simulink model "TPEtape3simulink"  (R2025b)
settings: Solver=VariableStepAuto  StartTime=0.0  StopTime=86400  RelTol=1e-3
libraries: cstblocks x2
settings Model: Creator=dayan  LastModifiedBy=dayan

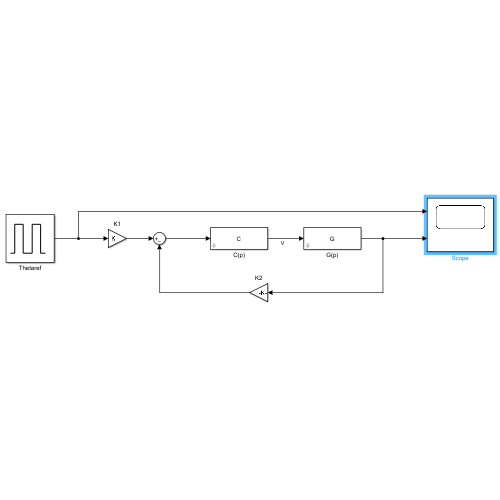
[thumbnail: Simulink's stored preview of the top-level diagram]
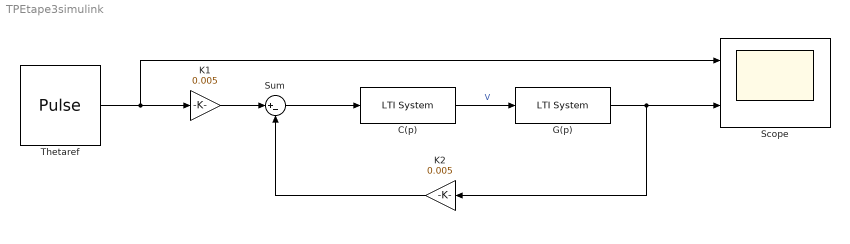
== system TPEtape3simulink ==
  C(p) : cstblocks/LTI System  sys=C  IC=[]  PadeOrder=0
  G(p) : cstblocks/LTI System  sys=G  IC=[]  PadeOrder=0
  K1 : Gain  Gain=0.005
  K2 : Gain  Gain=0.005
  Scope : Scope  NumInputPorts=2
      settings: ActiveDisplayYMinimum=-171.32921559343509  ActiveDisplayYMaximum=1352.3699128437149
  Sum : Sum  Inputs=|+-
  Thetaref : DiscretePulseGenerator  PulseType=Time based  Amplitude=1200  Period=15260  PulseWidth=90  SampleTime=15.26
  wires:
  C(p)/1 -> G(p)/1  "V"
  K1/1 -> Sum/1
  Sum/1 -> C(p)/1
  K2/1 -> Sum/2
  G(p)/1 -> Scope/2, K2/1
  Thetaref/1 -> Scope/1, K1/1
